simulink model "VF"  (R2023b)
settings: Solver=FixedStepAuto  StartTime=0.0  StopTime=2  FixedStep=1e-4  MaxStep=0.0001  RelTol=1e-3
values from neighbouring files (symbols this model uses):
  Pn = 4.0    [VF.sldd]
  Udc = 24.0    [VF.sldd]
libraries: mcbplantlib x1, autolibpmsmexterior x1
settings Model: DataDictionary=VF.sldd  Creator=00033411  LastModifiedBy=00033411
settings OptimizationCC: DefaultParameterBehavior=Inlined  UseDivisionForNetSlopeComputation=on  GainParamInheritBuiltInType=on  UseFloatMulNetSlope=on  InlineInvariantSignals=on  PassReuseOutputArgsAs=Individual arguments  ZeroExternalMemoryAtStartup=off  ZeroInternalMemoryAtStartup=off  NoFixptDivByZeroProtection=on  EfficientFloat2IntCast=on  LifeSpan=1  OptimizeBlockOrder=speed  DifferentSizesBufferReuse=on  EfficientTunableParamExpr=on
settings DebuggingCC: ParameterPrecisionLossMsg=none  ParameterTunabilityLossMsg=error
settings HardwareCC: ProdBitPerPointer=32  ProdBitPerSizeT=32  ProdBitPerPtrDiffT=32  ProdLargestAtomicInteger=Long  ProdLargestAtomicFloat=Double  ProdWordSize=32  ProdLongLongMode=on  ProdHWDeviceType=ARM Compatible->ARM Cortex-M
settings SFSimCC: MATLABDynamicMemAlloc=off
settings RTWCC: Description=Embedded Coder  SystemTargetFile=ert.tlc  TemplateMakefile=ert_default_tmf  GenerateReport=on  LaunchReport=on
settings CodeAppCC: ForceParamTrailComments=on  IgnoreCustomStorageClasses=off  OperatorAnnotations=on  SimulinkDataObjDesc=on  SFDataObjDesc=on  CustomSymbolStrGlobalVar=rt$N$M  CustomSymbolStrType=$N$M  CustomSymbolStrFcn=$N$M$F  CustomSymbolStrMacro=$N$M  InsertBlockDesc=on
settings ERTTargetCC: TargetLangStandard=C99 (ISO)  CodeReplacementLibrary=ARM Cortex-M  GenerateSampleERTMain=on  IncludeMdlTerminateFcn=off  CombineSignalStateStructs=on  SupportAbsoluteTime=off  SupportComplex=off  SupportNonInlinedSFcns=on  InlinedParameterPlacement=NonHierarchical  ERTCustomFileTemplate=example_file_process.tlc  ERTFilePackagingFormat=CompactWithDataFile

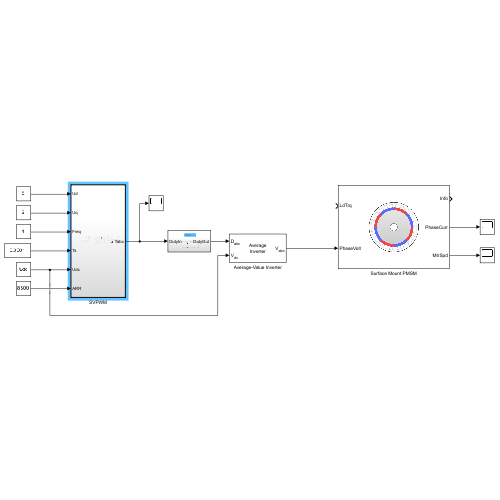
[thumbnail: Simulink's stored preview of the top-level diagram]
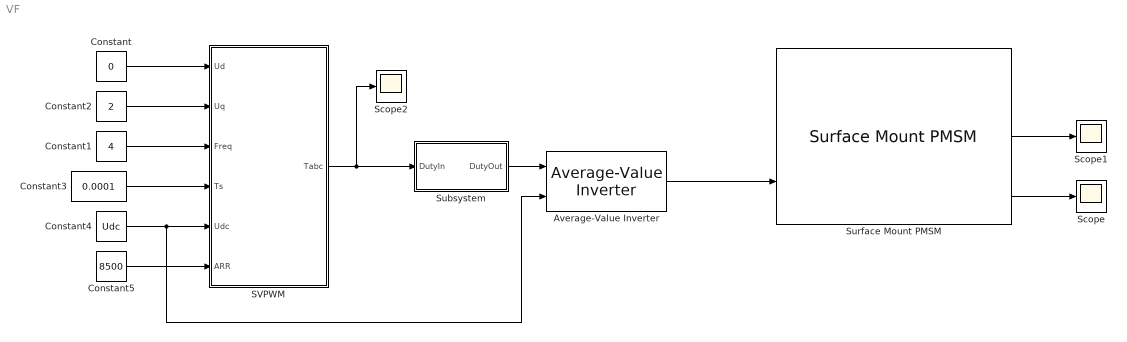
== system VF ==
  Average-Value Inverter : mcbplantlib/Average-Value Inverter
      settings: LibrarySourceBlock=mcblib/Electrical Systems/Inverters/Average-Value Inverter
  Constant : Constant  Value=0
  Constant1 : Constant  Value=4
  Constant2 : Constant  Value=2
  Constant3 : Constant  Value=0.0001
  Constant4 : Constant  Value=Udc
  Constant5 : Constant  Value=8500
  SVPWM : Subsystem  TreatAsAtomicUnit=on
  Scope : Scope
  Scope1 : Scope
  Scope2 : Scope
  Subsystem : Subsystem
  Surface Mount PMSM : autolibpmsmexterior/Surface Mount PMSM  port_config=Torque  sim_type=Discrete  Ts=1e-4  P=Pn  Rs=Rs  Ldq_=L  KConstText=Back-emf constant (Ke):  lambda_pm=3.59  Ke=Ke  Kt=1.323  mechanical=[1.55e-6, 3.86e-6, 0]  idq0=[0 0]  theta_init=0  omega_init=0  KConst=3.59  lambda_pm_calc=0.0049482  RefBlkName='autolibpmsmexterior/Surface Mount PMSM'  aMode=5  Ldq="[0.0017      0.0017]"
  wires:
  Constant/1 -> SVPWM/1(Ud)
  Constant1/1 -> SVPWM/3(Freq)
  Constant2/1 -> SVPWM/2(Uq)
  Constant3/1 -> SVPWM/4(Ts)
  Constant4/1 -> Average-Value Inverter/2, SVPWM/5(Udc)
  Constant5/1 -> SVPWM/6(ARR)
  Average-Value Inverter/1 -> Surface Mount PMSM/2
  SVPWM/1(Tabc) -> Subsystem/1(DutyIn), Scope2/1
  Surface Mount PMSM/2 -> Scope1/1
  Surface Mount PMSM/3 -> Scope/1
  Subsystem/1(DutyOut) -> Average-Value Inverter/1

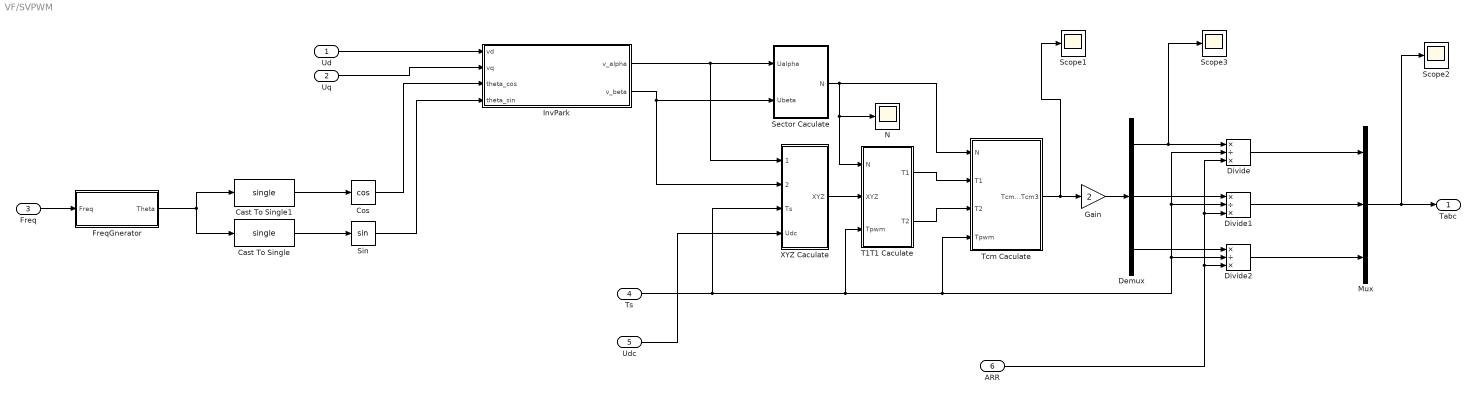
== system VF/SVPWM ==
  Ud : Inport
  Uq : Inport  Port=2
  Freq : Inport  Port=3
  Ts : Inport  Port=4
  Udc : Inport  Port=5
  ARR : Inport  Port=6
  Cast To Single : DataTypeConversion  OutDataTypeStr=single  SaturateOnIntegerOverflow=off  RndMeth=Floor
  Cast To Single1 : DataTypeConversion  OutDataTypeStr=single  SaturateOnIntegerOverflow=off  RndMeth=Floor
  Cos : Trigonometry  Operator=cos
  Demux : Demux  Outputs=3
  Divide : Product  Inputs=*/*
  Divide1 : Product  Inputs=*/*
  Divide2 : Product  Inputs=*/*
  FreqGnerator : Subsystem
  Gain : Gain  Gain=2
  InvPark : MATLAB Function  TreatAsAtomicUnit=on
  Mux : Mux  Inputs=3
  N : Scope
  Scope1 : Scope
  Scope2 : Scope
  Scope3 : Scope
  Sector Caculate : Subsystem
  Sin : Trigonometry
  T1T1 Caculate : Subsystem
  Tcm Caculate : Subsystem
  XYZ Caculate : Subsystem
  Tabc : Outport
  wires:
  Tcm Caculate/1(Tcm1 Tcm2 Tcm3) -> Gain/1, Scope1/1
  Divide1/1 -> Mux/2
  T1T1 Caculate/1(T1) -> Tcm Caculate/2(T1)
  Divide/1 -> Mux/1
  Cast To Single1/1 -> Cos/1
  ARR/1 -> Divide2/3, Divide1/3, Divide/3
  Cos/1 -> InvPark/3(theta_cos)
  Sector Caculate/1("N ") -> Tcm Caculate/1(N), N/1, T1T1 Caculate/1(N)
  Cast To Single/1 -> Sin/1
  T1T1 Caculate/2(T2) -> Tcm Caculate/3(T2)
  InvPark/2(v_beta) -> XYZ Caculate/2(Ubeta), Sector Caculate/2(Ubeta)
  InvPark/1(v_alpha) -> XYZ Caculate/1(Ualpha), Sector Caculate/1(Ualpha)
  XYZ Caculate/1(XYZ) -> T1T1 Caculate/2(XYZ)
  Gain/1 -> Demux/1
  Mux/1 -> Scope2/1, Tabc/1
  Divide2/1 -> Mux/3
  Demux/1 -> Scope3/1, Divide/1
  Demux/3 -> Divide2/1
  Demux/2 -> Divide1/1
  Sin/1 -> InvPark/4(theta_sin)
  FreqGnerator/1(Theta) -> Cast To Single/1, Cast To Single1/1
  Ud/1 -> InvPark/1(vd)
  Uq/1 -> InvPark/2(vq)
  Ts/1 -> Divide2/2, Divide1/2, Divide/2, Tcm Caculate/4(Tpwm), T1T1 Caculate/3(Tpwm), XYZ Caculate/3(Ts)
  Freq/1 -> FreqGnerator/1(Freq)
  Udc/1 -> XYZ Caculate/4(Udc)

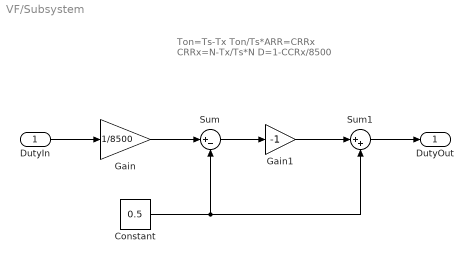
== system VF/Subsystem ==
  note: Ton=Ts-Tx Ton/Ts*ARR=CRRx
      | CRRx=N-Tx/Ts*N
      | D=1-CCRx/8500
  DutyIn : Inport
  Constant : Constant  Value=0.5  SampleTime=-1
  Gain : Gain  Gain=1/8500  ParamDataTypeStr=single
  Gain1 : Gain  Gain=-1
  Sum : Sum  Inputs=|+-
  Sum1 : Sum  Inputs=|++
  DutyOut : Outport
  wires:
  Sum/1 -> Gain1/1
  Constant/1 -> Sum1/2, Sum/2
  DutyIn/1 -> Gain/1
  Gain1/1 -> Sum1/1
  Sum1/1 -> DutyOut/1
  Gain/1 -> Sum/1

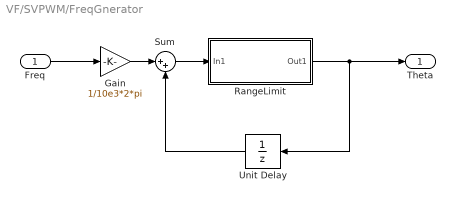
== system VF/SVPWM/FreqGnerator ==
  Freq : Inport
  Gain : Gain  Gain=1/10e3*2*pi
  RangeLimit : Subsystem
  Sum : Sum  Inputs=|++
  Unit Delay : UnitDelay  SampleTime=-1  HasFrameUpgradeWarning=on
  Theta : Outport
  wires:
  Freq/1 -> Gain/1
  RangeLimit/1(Out1) -> Unit Delay/1, Theta/1
  Gain/1 -> Sum/1
  Sum/1 -> RangeLimit/1(In1)
  Unit Delay/1 -> Sum/2

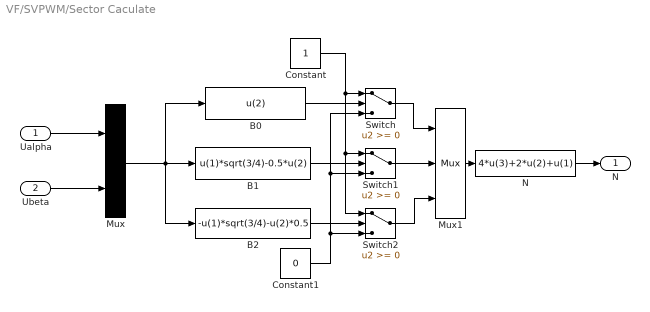
== system VF/SVPWM/Sector Caculate ==
  Ualpha : Inport
  Ubeta : Inport  Port=2
  B0 : Fcn  Expr=u(2)
  B1 : Fcn  Expr=u(1)*sqrt(3/4)-0.5*u(2)
  B2 : Fcn  Expr=-u(1)*sqrt(3/4)-u(2)*0.5
  Constant : Constant
  Constant1 : Constant  Value=0
  Mux : Mux  Inputs=2
  Mux1 : Mux  Inputs=3
  N : Fcn  Expr=4*u(3)+2*u(2)+u(1)
  Switch : Switch  SaturateOnIntegerOverflow=off  InputSameDT=off
  Switch1 : Switch  SaturateOnIntegerOverflow=off  InputSameDT=off
  Switch2 : Switch  SaturateOnIntegerOverflow=off  InputSameDT=off
  "N " : Outport
  wires:
  Switch2/1 -> Mux1/3
  Switch/1 -> Mux1/1
  Ualpha/1 -> Mux/1
  Ubeta/1 -> Mux/2
  Mux/1 -> B2/1, B1/1, B0/1
  B0/1 -> Switch/2
  B1/1 -> Switch1/2
  B2/1 -> Switch2/2
  Constant/1 -> Switch/1, Switch2/1, Switch1/1
  Constant1/1 -> Switch/3, Switch1/3, Switch2/3
  Switch1/1 -> Mux1/2
  Mux1/1 -> N/1
  N/1 -> "N "/1

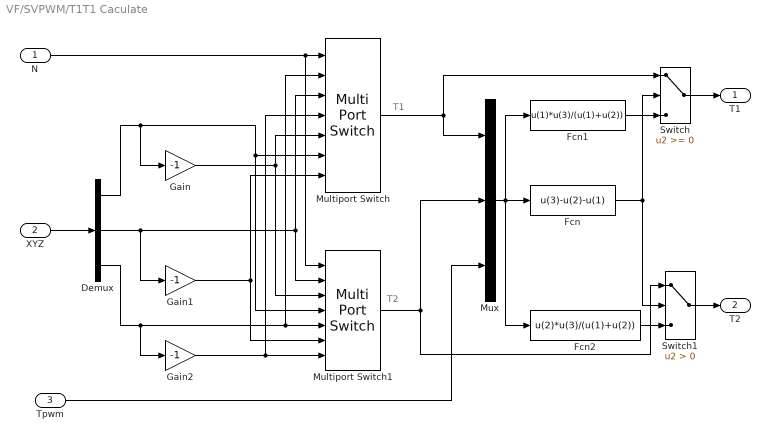
== system VF/SVPWM/T1T1 Caculate ==
  note: T1
  note: T2
  N : Inport
  XYZ : Inport  Port=2
  Tpwm : Inport  Port=3
  Demux : Demux  Outputs=3
  Fcn : Fcn  Expr=u(3)-u(2)-u(1)
  Fcn1 : Fcn  Expr=u(1)*u(3)/(u(1)+u(2))
  Fcn2 : Fcn  Expr=u(2)*u(3)/(u(1)+u(2))
  Gain : Gain  Gain=-1
  Gain1 : Gain  Gain=-1
  Gain2 : Gain  Gain=-1
  Multiport Switch : MultiPortSwitch  Inputs=6  SaturateOnIntegerOverflow=off  InputSameDT=off
  Multiport Switch1 : MultiPortSwitch  Inputs=6  SaturateOnIntegerOverflow=off  InputSameDT=off
  Mux : Mux  Inputs=3
  Switch : Switch  SaturateOnIntegerOverflow=off  InputSameDT=off
  Switch1 : Switch  Criteria=u2 > Threshold  SaturateOnIntegerOverflow=off  InputSameDT=off
  T1 : Outport
  T2 : Outport  Port=2
  wires:
  Tpwm/1 -> Mux/3
  XYZ/1 -> Demux/1
  Switch1/1 -> T2/1
  Switch/1 -> T1/1
  Fcn2/1 -> Switch1/3
  Fcn1/1 -> Switch/3
  Fcn/1 -> Switch/2, Switch1/2
  Mux/1 -> Fcn1/1, Fcn/1, Fcn2/1
  Multiport Switch/1 -> Switch/1, Mux/1
  Multiport Switch1/1 -> Switch1/1, Mux/2
  N/1 -> Multiport Switch/1, Multiport Switch1/1
  Demux/2 -> Multiport Switch/3, Multiport Switch1/2, Gain1/1
  Demux/3 -> Multiport Switch1/5, Multiport Switch/2, Gain2/1
  Demux/1 -> Multiport Switch/6, Multiport Switch1/4, Gain/1
  Gain/1 -> Multiport Switch1/3, Multiport Switch/5
  Gain2/1 -> Multiport Switch/4, Multiport Switch1/7
  Gain1/1 -> Multiport Switch1/6, Multiport Switch/7

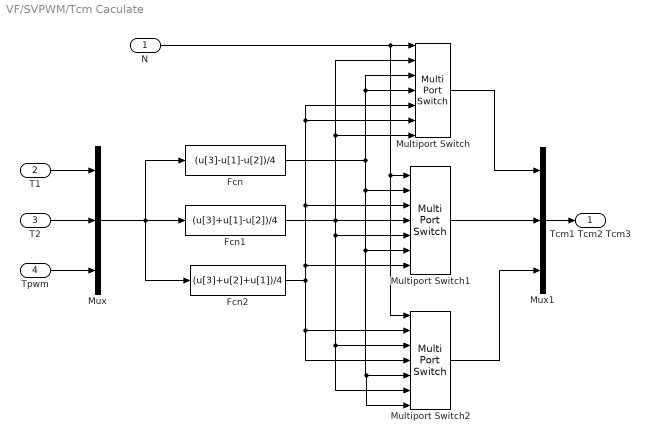
== system VF/SVPWM/Tcm Caculate ==
  N : Inport
  T1 : Inport  Port=2
  T2 : Inport  Port=3
  Tpwm : Inport  Port=4
  Fcn : Fcn  Expr=(u[3]-u[1]-u[2])/4
  Fcn1 : Fcn  Expr=(u[3]+u[1]-u[2])/4
  Fcn2 : Fcn  Expr=(u[3]+u[2]+u[1])/4
  Multiport Switch : MultiPortSwitch  Inputs=6  SaturateOnIntegerOverflow=off  InputSameDT=off
  Multiport Switch1 : MultiPortSwitch  Inputs=6  SaturateOnIntegerOverflow=off  InputSameDT=off
  Multiport Switch2 : MultiPortSwitch  Inputs=6  SaturateOnIntegerOverflow=off  InputSameDT=off
  Mux : Mux  Inputs=3
  Mux1 : Mux  Inputs=3
  Tcm1 Tcm2 Tcm3 : Outport
  wires:
  Mux/1 -> Fcn2/1, Fcn/1, Fcn1/1
  Tpwm/1 -> Mux/3
  T2/1 -> Mux/2
  T1/1 -> Mux/1
  Multiport Switch2/1 -> Mux1/3
  Multiport Switch1/1 -> Mux1/2
  Multiport Switch/1 -> Mux1/1
  Mux1/1 -> Tcm1 Tcm2 Tcm3/1
  Fcn/1 -> Multiport Switch/3, Multiport Switch/4, Multiport Switch1/6, Multiport Switch2/5, Multiport Switch2/7, Multiport Switch1/2
  Fcn1/1 -> Multiport Switch1/5, Multiport Switch2/3, Multiport Switch2/6, Multiport Switch1/4, Multiport Switch/7, Multiport Switch/2
  Fcn2/1 -> Multiport Switch/5, Multiport Switch/6, Multiport Switch1/3, Multiport Switch1/7, Multiport Switch2/2, Multiport Switch2/4
  N/1 -> Multiport Switch2/1, Multiport Switch1/1, Multiport Switch/1

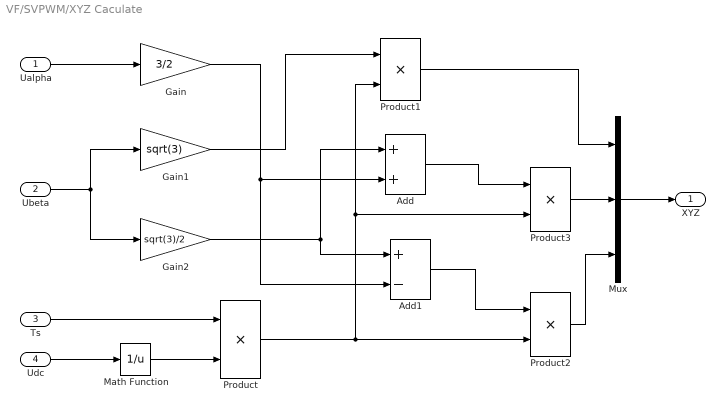
== system VF/SVPWM/XYZ Caculate ==
  Ualpha : Inport
  Ubeta : Inport  Port=2
  Ts : Inport  Port=3
  Udc : Inport  Port=4
  Add : Sum
  Add1 : Sum  Inputs=+-
  Gain : Gain  Gain=3/2
  Gain1 : Gain  Gain=sqrt(3)
  Gain2 : Gain  Gain=sqrt(3)/2
  Math Function : Math  Operator=reciprocal  SignedPower=on
  Mux : Mux  Inputs=3
  Product{,1..3} (4 alike) : Product  RndMeth=Zero
  XYZ : Outport
  wires:
  Mux/1 -> XYZ/1
  Product1/1 -> Mux/1
  Product3/1 -> Mux/2
  Product2/1 -> Mux/3
  Ualpha/1 -> Gain/1
  Ubeta/1 -> Gain2/1, Gain1/1
  Udc/1 -> Math Function/1
  Math Function/1 -> Product/2
  Ts/1 -> Product/1
  Gain1/1 -> Product1/1
  Product/1 -> Product2/2, Product1/2, Product3/2
  Gain/1 -> Add1/2, Add/2
  Gain2/1 -> Add/1, Add1/1
  Add1/1 -> Product2/1
  Add/1 -> Product3/1

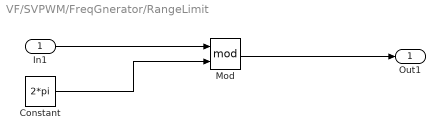
== system VF/SVPWM/FreqGnerator/RangeLimit ==
  In1 : Inport
  Constant : Constant  Value=2*pi
  Mod : Math  Operator=mod
  Out1 : Outport
  wires:
  In1/1 -> Mod/1
  Constant/1 -> Mod/2
  Mod/1 -> Out1/1

== matlab function VF/SVPWM/InvPark ==
  data: vd input; v_alpha output; vq input; theta_cos input; theta_sin input; v_beta output
function [v_alpha, v_beta] = InvPark_Voltage(vd, vq, theta_cos, theta_sin)
% ==============================
% 电压型 反Park变换
% dq旋转坐标系 → αβ静止坐标系
% 输入：
%   vd        : d轴电压（电流环PI输出）
%   vq        : q轴电压（电流环PI输出）
%   theta_cos : 电角度余弦 cosθ
%   theta_sin : 电角度正弦 sinθ
% 输出：
%   v_alpha   : α轴静止电压
%   v_beta    : β轴静止电压
% ==============================

% 反Park标准公式（电压/电流通用）
v_alpha = vd * theta_cos - vq * theta_sin;
v_beta  = vd * theta_sin + vq * theta_cos;
end
